simulink model "WheelSpeeds"  (R2024b)
settings: configuration reference "STM32H7_Config" (kept outside this file)
undefined symbols (not defined in the file): rGearboxRatio, rTyreRadius
settings Model: DataDictionary=Master_Dictionary.sldd  EnableAccessToBaseWorkspace=off  Creator=torni  LastModifiedBy=William
settings ConfigSetRef: SourceName=STM32H7_Config

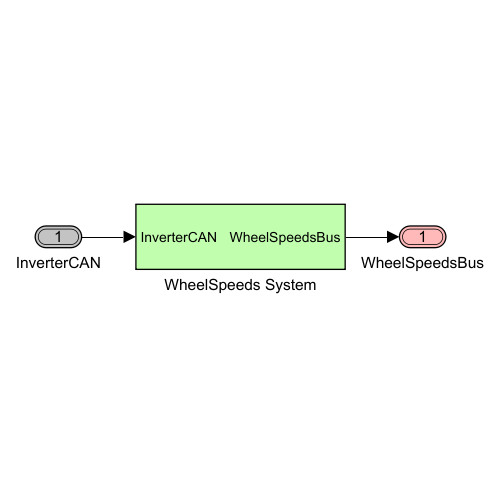
[thumbnail: Simulink's stored preview of the top-level diagram]
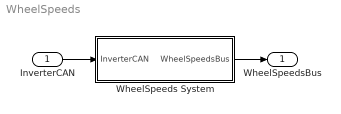
== system WheelSpeeds ==
  InverterCAN : Inport  OutDataTypeStr=Bus: CAN1_2Bus
  WheelSpeeds System : Subsystem
  WheelSpeedsBus : Outport  OutDataTypeStr=Bus: WheelSpeedsBus  VectorParamsAs1DForOutWhenUnconnected=off
  wires:
  InverterCAN/1 -> WheelSpeeds System/1(InverterCAN)
  WheelSpeeds System/1(WheelSpeedsBus) -> WheelSpeedsBus/1

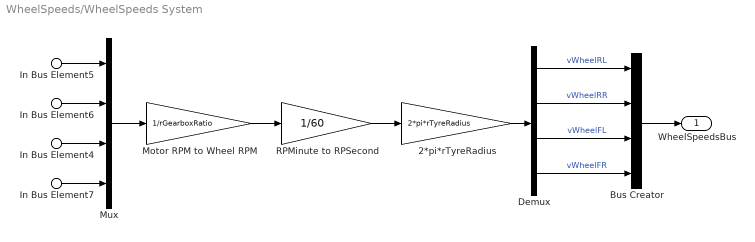
== system WheelSpeeds/WheelSpeeds System ==
  In Bus Element4 : Inport  PortName=InverterCAN  Element=InverterFLCANBus.nMotorFL
  In Bus Element5 : Inport  PortName=InverterCAN  Element=InverterRLCANBus.nMotorRL
  In Bus Element6 : Inport  PortName=InverterCAN  Element=InverterRRCANBus.nMotorRR
  In Bus Element7 : Inport  PortName=InverterCAN  Element=InverterFRCANBus.nMotorFR
  2*pi*rTyreRadius : Gain  Gain=2*pi*rTyreRadius
  Bus Creator : BusCreator  Inputs=4  OutDataTypeStr=Bus: WheelSpeedsBus
  Demux : Demux
  Motor RPM to Wheel RPM : Gain  Gain=1/rGearboxRatio
  Mux : Mux
  RPMinute to RPSecond : Gain  Gain=1/60
  WheelSpeedsBus : Outport  OutDataTypeStr=Bus: WheelSpeedsBus  VectorParamsAs1DForOutWhenUnconnected=off
  wires:
  Demux/1 -> Bus Creator/1  "vWheelRL"
  Demux/2 -> Bus Creator/2  "vWheelRR"
  Demux/4 -> Bus Creator/4  "vWheelFR"
  Demux/3 -> Bus Creator/3  "vWheelFL"
  In Bus Element5/1 -> Mux/1
  In Bus Element6/1 -> Mux/2
  In Bus Element4/1 -> Mux/3
  In Bus Element7/1 -> Mux/4
  RPMinute to RPSecond/1 -> 2*pi*rTyreRadius/1
  Mux/1 -> Motor RPM to Wheel RPM/1
  Motor RPM to Wheel RPM/1 -> RPMinute to RPSecond/1
  2*pi*rTyreRadius/1 -> Demux/1
  Bus Creator/1 -> WheelSpeedsBus/1
